simulink model "test_controlador_trolley"  (R2023b)
settings: Solver=FixedStepAuto  StartTime=0.0  StopTime=10  FixedStep=0.001  RelTol=1e-3
undefined symbols (not defined in the file or in its folder): r_td
libraries: robotcorelib x1
settings Model: Creator=Ferran  LastModifiedBy=Ferran
settings DebuggingCC: AlgebraicLoopMsg=none  ArtificialAlgebraicLoopMsg=none

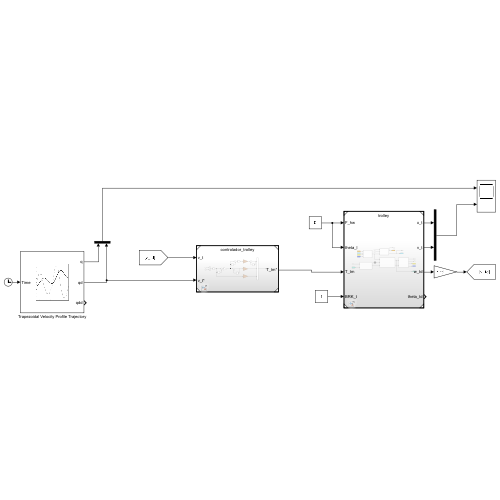
[thumbnail: Simulink's stored preview of the top-level diagram]
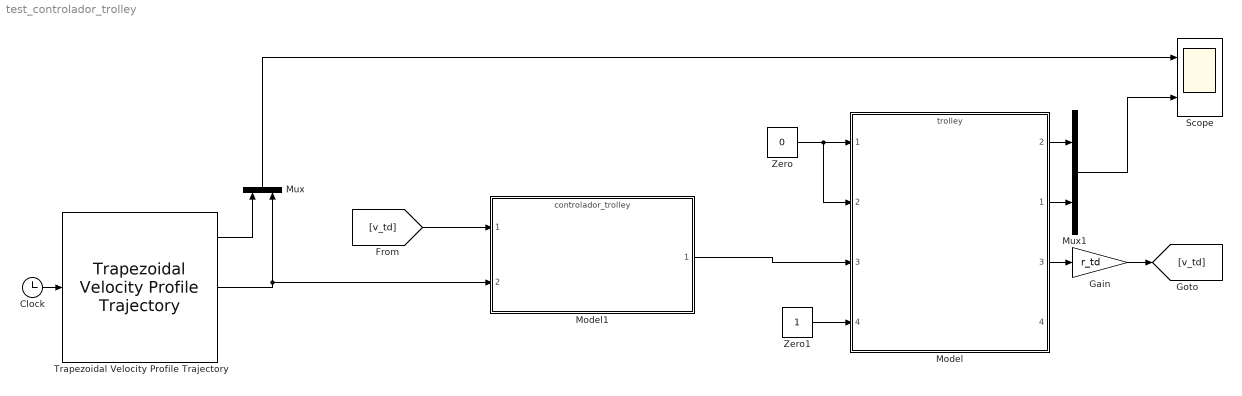
== system test_controlador_trolley ==
  Clock : Clock
  Gain : Gain  Gain=r_td
  Model : ModelReference  ModelNameDialog=trolley.slx  SimulationMode=Normal  ModelReferenceVersion=1.27
      settings: PortSchema="{\"entries\":[{\"content\":{\"sides\":[{\"content\":{\"connectorIds\":[\"In1\",\"In2\",\"In3\",\"In4\"]},\"type\":\"ConnectorPlacement.EquallySpacedRectSide\",\"uuid\":\"1b29c0b7-3c94-4f8d-80c7-b7c67fb71c78\"},{\"content\":{\"connectorIds\":[\"Out2\",\"Out1\",\"Out3\",\"Out4\"],\"side\":\"RIGHT\"},\"type\":\"ConnectorPlacement.EquallySpacedRectSide\",\"uuid\":\"0e621dc3-1b80-4463-b355-e1f568b8f818\"},{\"content\":{\"side\":\"TOP\"},\"type\":\"ConnectorPlacement.EquallySpacedRectSide\",\"uuid\":\"071687c5-a0c6-43a6-aaac-1f68313cffd7\"}]},\"type\":\"ConnectorPlacement.EquallySpacedConnector\",\"uuid\":\"1fb9a635-ae67-4097-bbc1-74c46d02297b\"}],\"packageUris\":[\"http://schema.mathworks.com/mf0/Connector/R2020b\"],\"version\":\"1.0\"}"
  Model1 : ModelReference  ModelNameDialog=controlador_trolley.slx  SimulationMode=Normal  ModelReferenceVersion=2.16
  Mux : Mux  Inputs=2
  Mux1 : Mux  Inputs=2
  Scope : Scope  NumInputPorts=2
  Trapezoidal Velocity Profile Trajectory : robotcorelib/Trapezoidal Velocity Profile Trajectory  WaypointSource=Internal  Waypoints=[0, 1]  NumParams=1  Parameter1=Peak Velocity  Parameter2=End Time  ParameterSource=Internal  PeakVelocity=[ 1 ]  Acceleration=[ 1; 2 ]  EndTime=[ 1]  AccelTime=[ 1; 2 ]  SimulateUsing=Interpreted execution
  Zero : Constant  Value=0  OutDataTypeStr=Inherit: Inherit via back propagation
  Zero1 : Constant  OutDataTypeStr=Inherit: Inherit via back propagation
  wires:
  Model/1 -> Mux1/2
  Model/3 -> Gain/1
  [v_td] -> Model1/1
  Model/2 -> Mux1/1
  Mux/1 -> Scope/1
  Clock/1 -> Trapezoidal Velocity Profile Trajectory/1
  Mux1/1 -> Scope/2
  Zero/1 -> Model/2, Model/1
  Trapezoidal Velocity Profile Trajectory/2 -> Model1/2, Mux/2
  Zero1/1 -> Model/4
  Gain/1 -> [v_td]
  Trapezoidal Velocity Profile Trajectory/1 -> Mux/1
  Model1/1 -> Model/3
